simulink subsystem "IR_LED_Pattern"  (R2024a)
settings: Solver=VariableStepAuto  StartTime=0.0  StopTime=10.0  RelTol=1e-3
undefined symbols (not defined in the file or in its folder): IR_LED_PERIOD
settings Model: Creator=JesseJabezArendse  LastModifiedBy=Chris Scheepers
settings RTWCC: GPUComputeCapability=3.5

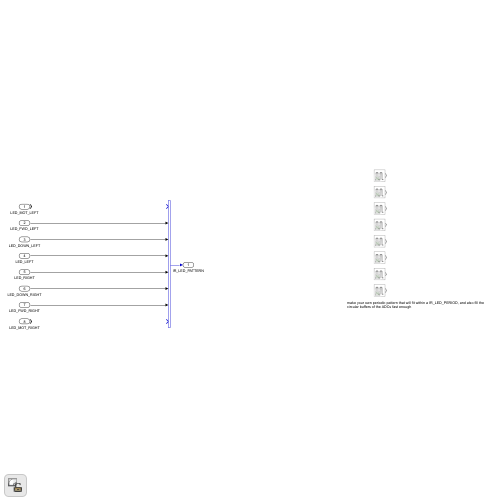
[thumbnail: Simulink's stored preview of the top-level diagram]
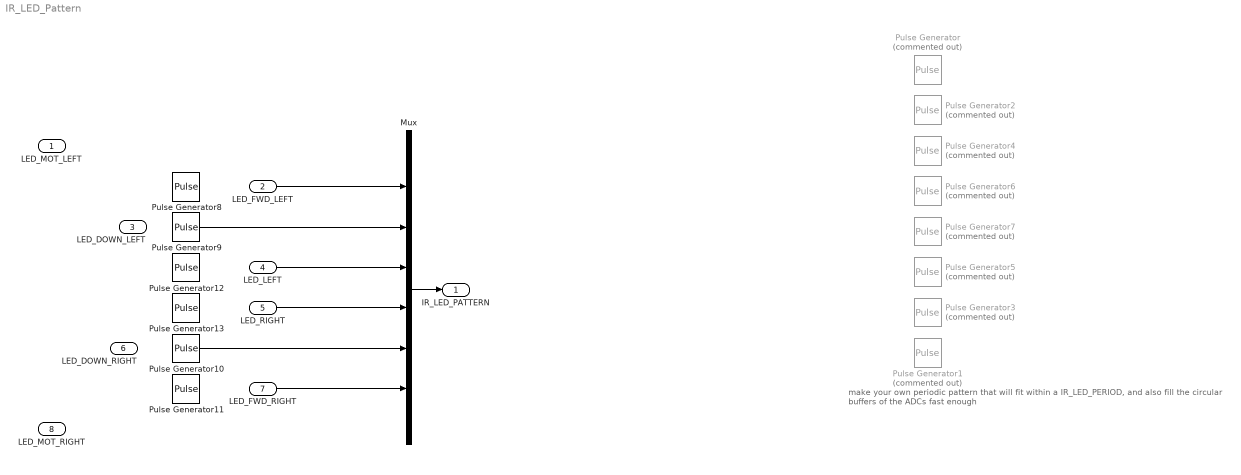
== system IR_LED_Pattern ==
  note: make your own periodic pattern that will fit within a IR_LED_PERIOD, and also fill the circular buffers of the ADCs fast enough
  LED_MOT_LEFT : Inport
  LED_FWD_LEFT : Inport  Port=2
  LED_DOWN_LEFT : Inport  Port=3
  LED_LEFT : Inport  Port=4
  LED_RIGHT : Inport  Port=5
  LED_DOWN_RIGHT : Inport  Port=6
  LED_FWD_RIGHT : Inport  Port=7
  LED_MOT_RIGHT : Inport  Port=8
  Mux : Mux  Inputs=8
  Pulse Generator : DiscretePulseGenerator  Commented=on  PulseType=Time based  Period=0.2  PulseWidth=25
  Pulse Generator1 : DiscretePulseGenerator  Commented=on  PulseType=Time based  Period=0.2  PulseWidth=25
  Pulse Generator{8..11} (4 alike) : DiscretePulseGenerator  PulseType=Time based  Period=IR_LED_PERIOD  PulseWidth=50
  Pulse Generator12 : DiscretePulseGenerator  PulseType=Time based  Period=IR_LED_PERIOD  PulseWidth=50  PhaseDelay=IR_LED_PERIOD*0.5
  Pulse Generator13 : DiscretePulseGenerator  PulseType=Time based  Period=IR_LED_PERIOD  PulseWidth=50  PhaseDelay=IR_LED_PERIOD*0.5
  Pulse Generator2 : DiscretePulseGenerator  Commented=on  PulseType=Time based  Period=0.2  PulseWidth=25  PhaseDelay=0.05
  Pulse Generator3 : DiscretePulseGenerator  Commented=on  PulseType=Time based  Period=0.2  PulseWidth=25  PhaseDelay=0.05
  Pulse Generator4 : DiscretePulseGenerator  Commented=on  PulseType=Time based  Period=0.2  PulseWidth=25  PhaseDelay=0.1
  Pulse Generator5 : DiscretePulseGenerator  Commented=on  PulseType=Time based  Period=0.2  PulseWidth=25  PhaseDelay=0.1
  Pulse Generator6 : DiscretePulseGenerator  Commented=on  PulseType=Time based  Period=0.2  PulseWidth=25  PhaseDelay=0.15
  Pulse Generator7 : DiscretePulseGenerator  Commented=on  PulseType=Time based  Period=0.2  PulseWidth=25  PhaseDelay=0.15
  IR_LED_PATTERN : Outport
  wires:
  Mux/1 -> IR_LED_PATTERN/1
  Pulse Generator9/1 -> Mux/3
  Pulse Generator10/1 -> Mux/6
  LED_FWD_LEFT/1 -> Mux/2
  LED_LEFT/1 -> Mux/4
  LED_RIGHT/1 -> Mux/5
  LED_FWD_RIGHT/1 -> Mux/7
